simulink model "Discrete_Time_Sim_With_Noise"  (R2024b)
settings: Solver=FixedStepAuto  StartTime=0.0  StopTime=10  FixedStep=0.001  RelTol=1e-3
undefined symbols (not defined in the file or in its folder): DiscIntNeverNeededParam, dspblkCoreblockFVToolHelper, gcbh
libraries: simulink x12, sharedTrackingLibrary x1
(part 1 of 4)
settings Model: Creator=BU  LastModifiedBy=BU

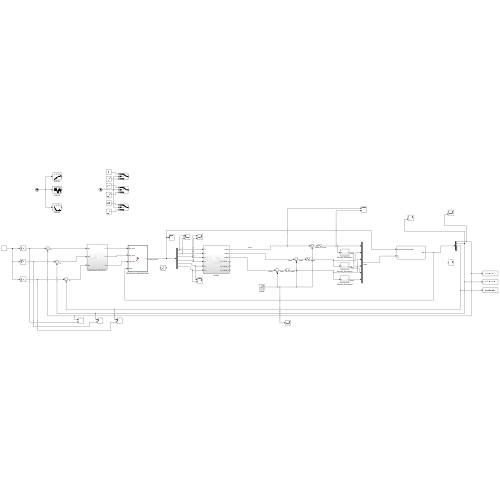
[thumbnail: Simulink's stored preview of the top-level diagram]
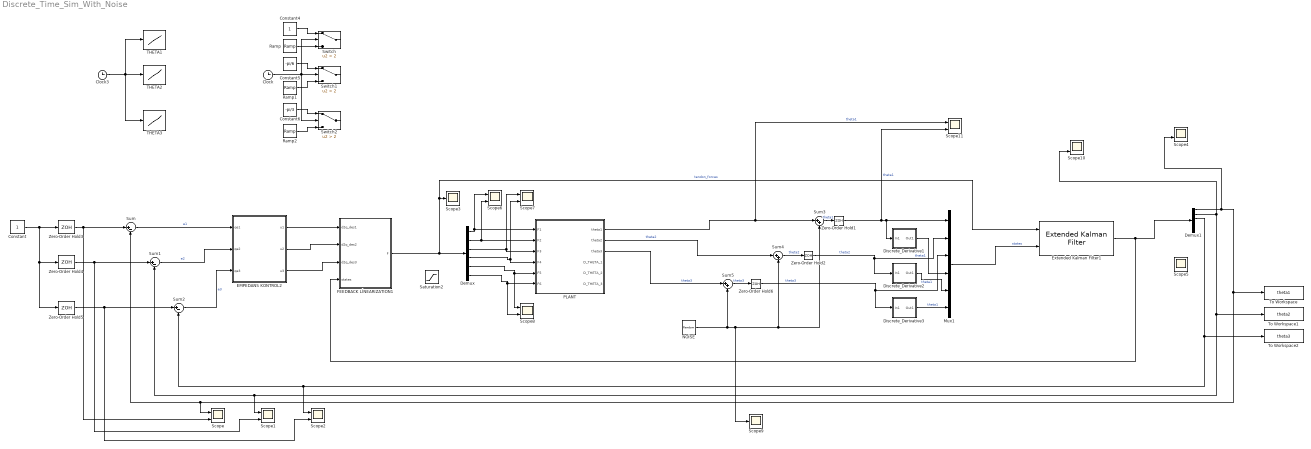
== system Discrete_Time_Sim_With_Noise ==
  Clock : Clock
  Clock3 : Clock
  Constant : Constant
  Constant4 : Constant
  Constant5 : Constant  Value=-pi/6
  Constant6 : Constant  Value=-pi/3
  Demux : Demux  Outputs=6
  Demux1 : Demux  Outputs=6
  Discrete_Derivative1 : Subsystem
  Discrete_Derivative2 : Subsystem
  Discrete_Derivative3 : Subsystem
  EMPEDANS KONTROL2 : Subsystem
  Extended Kalman Filter1 : sharedTrackingLibrary/Extended Kalman Filter  StateTransitionFcn=myStateTransitionFcn  HasStateTransitionJacobianFcn=off  StateTransitionJacobianFcn=0  HasAdditiveProcessNoise=Additive  ProcessNoise=diag([1e-7, 1e-7, 1e-7, 1e-7, 1e-7, 1e-7]);  HasTimeVaryingProcessNoise=off  HasStateTransitionFcnExtraArgument=1  InitialState=[0; 0; 0; 0; 0; 0]  InitialStateCovariance=[1e-6; 1e-6; 1e-6; 1e-6; 1e-6; 1e-6];  MeasurementFcn1=myMeasurementFcn  HasMeasurementJacobianFcn1=off  HasMeasurementEnablePort1=off  HasAdditiveMeasurementNoise1=Additive  MeasurementNoise1=[1e-1; 1e-1; 1e-1; 1e-1; 1e-1; 1e-1];  HasTimeVaryingMeasurementNoise1=off  HasMeasurementFcnExtraArgument1=0  HasMeasurementWrapping1=off  MeasurementFcn2=myMeasurementFcn  HasMeasurementJacobianFcn2=off  HasMeasurementEnablePort2=off  HasAdditiveMeasurementNoise2=Additive  MeasurementNoise2=1  HasTimeVaryingMeasurementNoise2=off  HasMeasurementFcnExtraArgument2=0  HasMeasurementWrapping2=off  MeasurementFcn3=myMeasurementFcn  HasMeasurementJacobianFcn3=off  HasMeasurementEnablePort3=off  HasAdditiveMeasurementNoise3=Additive  MeasurementNoise3=1  HasTimeVaryingMeasurementNoise3=off  HasMeasurementFcnExtraArgument3=0  HasMeasurementWrapping3=off  MeasurementFcn4=myMeasurementFcn  HasMeasurementJacobianFcn4=off  HasMeasurementEnablePort4=off  HasAdditiveMeasurementNoise4=Additive  MeasurementNoise4=1  HasTimeVaryingMeasurementNoise4=off  HasMeasurementFcnExtraArgument4=0  HasMeasurementWrapping4=off  MeasurementFcn5=myMeasurementFcn  HasMeasurementJacobianFcn5=off  HasMeasurementEnablePort5=off  HasAdditiveMeasurementNoise5=Additive  MeasurementNoise5=1  HasTimeVaryingMeasurementNoise5=off  HasMeasurementFcnExtraArgument5=0  HasMeasurementWrapping5=off  EnableMultirate=off  StateTransitionFcnSampleTime=1  MeasurementFcn1SampleTime=1  MeasurementFcn2SampleTime=1  MeasurementFcn3SampleTime=1  MeasurementFcn4SampleTime=1  MeasurementFcn5SampleTime=1  UseCurrentEstimator=on  OutputStateCovariance=off  DataType=double  SampleTime=0.001  NumberOfMeasurements=1
      settings: LibrarySourceBlock=slident/Estimators/Extended Kalman Filter
  FEEDBACK LİNEARIZATION1 : MATLAB Function  TreatAsAtomicUnit=on
  Mux1 : Mux  Inputs=6
  NOİSE : RandomNumber  Variance=6e-6  SampleTime=0.001
  PLANT : Subsystem
  Ramp : simulink/Sources/Ramp  slope=0.5  start=0  InitialOutput=0
  Ramp1 : simulink/Sources/Ramp  slope=-pi/12  start=0  InitialOutput=0
  Ramp2 : simulink/Sources/Ramp  slope=-pi/6  start=0  InitialOutput=0
  Saturation2 : Saturate  UpperLimit=7  LowerLimit=-7
  Scope{,1..2,4,6..8,10..11} (9 alike) : Scope  NumInputPorts=2
  Scope3 : Scope
  Scope5 : Scope
  Scope9 : Scope
  Sum : Sum  Inputs=|+-
  Sum1 : Sum  Inputs=|+-
  Sum2 : Sum  Inputs=|+-
  Sum3 : Sum  Inputs=|++
  Sum4 : Sum  Inputs=|++
  Sum5 : Sum  Inputs=|++
  Switch : Switch  Criteria=u2 > Threshold  Threshold=2  SaturateOnIntegerOverflow=off  InputSameDT=off
  Switch1 : Switch  Criteria=u2 > Threshold  Threshold=2  SaturateOnIntegerOverflow=off  InputSameDT=off
  Switch2 : Switch  Criteria=u2 > Threshold  Threshold=2  SaturateOnIntegerOverflow=off  InputSameDT=off
  THETA1 : Lookup_n-D  NumberOfTableDimensions=1  BreakpointsForDimension1=[0:0.02649:20]  Table="[3.6739403974420595e-17  0.0018373747386941153  0.031104117726482236  0.018742775985835458  0.03582520263747096  0.04592374641467687  0.052359865334245005  0.024058789434421298  0.0371846744639253  0.03766299609142134  0.04053395039223553  0.05419725229851646  0.03858245137367349  0.06940555854089034  0.07349874804657569  0.06036247150750728  0.05603574389361684  0.060203800337469145  0.05742707768917204  0.08742903616174802  0.08902502526928899  0.08910383733839858  0.06737978568977998  0.07977308569010028  0.07440905071740662  0.12217303541401832  0.09094232893350204  0.08904496692572651  0.10747616617119161  0.10938974392795553  0.13962632793396143  0.1083956214534407  0.18488795370701283  0.12080807257958151  0.19198621771937807  0.20053536868258393  0.13958180389913316  0.15159411331235176  0.21221713449958643  0.20813879967607254  0.1559933516267367  0.13924408208160471  0.15768074798413845  0.14168292749125272  0.22330906860945512  0.15983604373103352  0.16455025763473308  0.17031601131911764  0.23328736831901986  0.16908920173142786  0.24223952083150546  0.16676295276355868  0.2460466761118888  0.2427442300425048  0.2486574882599835  0.2524091142547836  0.26497062155526524  0.2686031710582675  0.2501965607304947  0.26676047671265896  0.2643551632848289  0.19274332249535645  0.2738619349890345  0.28220592554301155  0.28811598890932444  0.2734154158379111  0.19658209835701151  0.21602121918276904  0.2672822987058359  0.3286381062553793  0.31016072985042253  0.3333562023023043  0.3206007450683914  0.24027818402917203  0.26820372925417835  0.2671750205501374  0.3316125578789242  0.3426470130069342  0.3512794501726035  0.35378674308527575  0.34906585039886256  0.3602220148407348  0.334007825546644  0.35850389060191834  0.36346154149840965  0.3499372161164522  0.27940999409903805  0.3615110009749353  0.2829285466528819  0.28907124992067035  0.2958562209487426  0.37063784854548126  0.38431676246130947  0.3872502136853321  0.38783712884126237  0.3085945485814749  0.2961223513979233  0.31466855250366454  0.38909946387464134  0.3798718789620668  0.4007313511201461  0.4014257279586968  0.38565996627791466  0.330166531071065  0.33344993261761385  0.3108624823799387  0.3352853086354352  0.40657748147216466  0.34998446799647454  0.3343689689304545  0.4014257279586976  0.4111813198409137  0.3988981447289421  0.4186382947143397  0.40142572795869536  0.41887902047864184  0.4290229802606445  0.41781912282973876  0.41795816369666855  0.43746763932430155  0.41493598188809466  0.43603007682123895  0.41732493944380256  0.34440344919783417  0.42938623750992094  0.45298201367972535  0.4288419913470435  0.3677411229875971  0.43758514195346915  0.3865802197767727  0.3751084506612871  0.44814429494692254  0.3720896409650807  0.4525537516630718  0.45581996404987013  0.46350881524855264  0.3868228290174442  0.46007677244678846  0.47338681502372737  0.4712388980384691  0.4493903916162998  0.4642709337838176  0.4032631026973869  0.4685622431028752  0.3883857325472519  0.46719629998405016  0.4795595869316255  0.41992086739321355  0.3914676248964888  0.40759533432809686  0.48633741377695394  0.503361410251195  0.4837780015498778  0.4884893851013152  0.41753664465676027  0.4085774671942687  0.4315817277722004  0.42719707263790824  0.5026342919632628  0.5125437672769803  0.44002440524952796  0.4333772620748816  0.5105491774179737  0.5281996949991661  0.4886921905584105  0.4282797975188503  0.5173518691902903  0.5238681952025085  0.5278284238409199  0.5288725340894371  0.5416647490392732  0.5149332000522006  0.5502478095136083  0.5462177778009292  0.5402498088439542  0.5286973749476239  0.45219733563073633  0.5333967879492966  0.5410820534657627  0.4704351055583119  0.5421823655200836  0.5559404870228405  0.48551809760352327  0.5480768236319203  0.5574563364291668  0.5719520739146396  0.5718223517553729  0.5747046356092969  0.5591900066960385  0.5579012852080848  0.5530351144405614  0.5664360138663578  0.566709099544408  0.5816224503929176 ...(+11127 chars)];"  InternalRulePriority=Speed  RndMeth=Simplest
  THETA2 : Lookup_n-D  NumberOfTableDimensions=1  BreakpointsForDimension1=[0:0.02649:20]  Table="[0.0  0.03490658503988885  -0.033284041948025575  0.024108973093034097  0.017453292519947913  0.010897133595376871  2.580956827951785e-08  0.05801510497744568  0.04868897935829344  0.05235987755982642  0.060690073963622776  0.03490658503990476  0.06981317007977231  0.024238413989330437  0.014730566219418576  0.05579073535311509  0.06981317007977231  0.06823361310456687  0.08130478950558964  0.028160994381164636  0.03194749988012217  0.034906585039914305  0.08472703296472568  0.07144632904991825  0.08726646259971634  2.580956827951785e-08  0.06981317007977549  0.08192340488382562  0.05235987755983278  0.05540554109194949  2.580956827951785e-08  0.06981317007978505  -0.08840686306026094  0.056301906362856584  -0.08726646259972015  -0.09992958834775573  0.04124423707398681  0.024523948301493594  -0.10278030666584669  -0.08493047048957507  0.0330576678310699  0.07509376311585307  0.044753552033083295  0.08238435334413935  -0.09053757172286077  0.052359877559807325  0.04559052981096805  0.04183361289751157  -0.08806346617828203  0.05457713814060981  -0.10020250825383402  0.06585773908739219  -0.09503207893317432  -0.08382912684246552  -0.0886095062350847  -0.08877482543867116  -0.11289958939038655  -0.11400494326389625  -0.06780086460973182  -0.09787633235095192  -0.08494579017009243  0.07259786120584893  -0.09502044892588707  -0.10858388920763397  -0.11716142564727819  -0.07797060352501026  0.0872664625997125  0.08623656651485352  0.008941650029711387  -0.12003519103250365  -0.07443881028729186  -0.12005690683677152  -0.08711768024630258  0.08609866483557414  0.037707101369440575  0.04564547046169879  -0.08726646259972015  -0.10740555498876758  -0.12175208995592679  -0.12075780610488446  -0.10471975511965279  -0.12431198461645662  -0.06124914974178794  -0.10914281092122118  -0.11751340501827023  -0.08264071659361362  0.06996856329094929  -0.09923579646961392  0.06981317007976753  0.06356008523867811  0.059060910667330074  -0.09563230456995794  -0.120231530929497  -0.1233688014218704  -0.12118747138531023  0.05273873482906122  0.08047001912219476  0.04667516779941028  -0.10697141125366606  -0.08244410112317954  -0.12423265131075169  -0.12217304763960532  -0.0839214967334022  0.03814885382421918  0.034906585039895216  0.08535061346156758  0.039753719555991836  -0.10723463591055922  0.017453292519897023  0.05235987755983278  -0.08726646259972015  -0.10420225604982192  -0.07319022629209936  -0.11164835857706268  -0.06981317007977231  -0.10471975511966554  -0.12268815644386528  -0.09427459346404958  -0.09243646265768085  -0.1304306398657574  -0.07894393826895223  -0.12050390133646655  -0.07656286796138893  0.08061183608047065  -0.08894014674562721  -0.1357335445848138  -0.07816767295833149  0.054119332737865365  -0.08935408926939761  0.02199468753231221  0.05029869437163041  -0.10100975249936778  0.06255747691272129  -0.10489102534646705  -0.10819821457663435  -0.11931485080023811  0.04600742129117378  -0.1061216956455849  -0.1308529653505546  -0.1221730476396035  -0.07202008470981623  -0.099462587755587  0.034906585039895216  -0.10009203093905035  0.07120370686977313  -0.08849603242699301  -0.11159991366826001  0.01842492915558315  0.08166734018060748  0.05474075805682762  -0.10779457600445713  -0.1411952409075954  -0.0946854051550396  -0.10105261328295449  0.052105244970079956  0.0805434765835345  0.039851461664634664  0.05120354563972951  -0.10572128681989593  -0.12333296158987568  0.03422551094635462  0.05191335639712643  -0.10740470199761225  -0.14150127587830474  -0.05235987755982642  0.07865865445022234  -0.090142570581727  -0.10009950108652808  -0.10559245849112399  -0.10486516636439701  -0.12910085175104827  -0.06839935798121312  -0.14041441654823544  -0.12793480610576502  -0.11190815237909614  -0.08442067718491744  0.08121382491144723  -0.08763734115108718  -0.09968809522423466  0.05255504521596442  -0.09395492969943792  -0.12070347296111478  0.0322100128957269  -0.09931879841590988  -0.11511469777161175 ...(+12333 chars)];"  InternalRulePriority=Speed  RndMeth=Simplest
  THETA3 : Lookup_n-D  NumberOfTableDimensions=1  BreakpointsForDimension1=[0:0.02649:20]  Table="[1.4901161157108252e-08  -0.08910383733841787  -0.0327266608183487  -0.12139156541861737  -0.17545154279702416  -0.19644722016959976  -0.19198623130335932  -0.21297358831144533  -0.2429532865017081  -0.2471025063307386  -0.27575694955529145  -0.2636367625378544  -0.282928546652879  -0.29435683650957045  -0.2802155319853704  -0.32559271709994325  -0.3352884242127084  -0.34660356994132824  -0.36562466995402293  -0.3512094795621464  -0.365318620428616  -0.3683565176575177  -0.3964529139337104  -0.4130188025391666  -0.4234749011162723  -0.4014257415426788  -0.4400081793323686  -0.45894769838861765  -0.45654201657006255  -0.47022790411891413  -0.4537856191025084  -0.49236805689220453  -0.41064035600573134  -0.49999589056138904  -0.4363323129985795  -0.4409449844737227  -0.5386185376319574  -0.5426372045326548  -0.4759559707525487  -0.4984541183652786  -0.5730234548965603  -0.6070369268961825  -0.603860027975918  -0.6254930087940876  -0.5254705785853191  -0.6136216492495379  -0.6115665154043974  -0.6223019984352975  -0.5553762763594051  -0.6425453603506759  -0.5521893867963389  -0.6514997123295901  -0.5786202639173261  -0.5865207699386508  -0.5963802950234814  -0.6086932480746661  -0.5971299914234329  -0.608383833312897  -0.6449079478992603  -0.6313963961402045  -0.6506482711532061  -0.7453067279996465  -0.6588070303615892  -0.6535875806338188  -0.6509201075604881  -0.6841370028713132  -0.7725407515151371  -0.8258565612959209  -0.8260026631137608  -0.7496549833411186  -0.7855006339413441  -0.7630780098437462  -0.7919884254602746  -0.8848822095029318  -0.8731428375217765  -0.888779144169965  -0.8203047484373329  -0.8112001111762953  -0.8054860133748054  -0.8177142363984913  -0.8377580409572819  -0.8293219759023509  -0.8748972677429  -0.851499671618741  -0.8480867284181834  -0.8781617377208543  -0.960243795588003  -0.8731404427033367  -0.9636069549306653  -0.9634965733573642  -0.9745090160740592  -0.8945974284335108  -0.8836771159897994  -0.8834732967214486  -0.8862415419139391  -0.9896518141284941  -1.0049109012380764  -0.9983888972810051  -0.9191732295989057  -0.9431996010767902  -0.9222705230472953  -0.9250245035569944  -0.9562369390423859  -1.031540500653129  -1.031581633415354  -1.0594382115993513  -1.0469907902092443  -0.9712946075794223  -1.0481161687941598  -1.067407254768076  -0.9948376736367662  -0.9876574720688799  -1.0151129729746031  -0.9963949906750376  -1.0297442586766548  -1.0122909661567079  -1.0044665246145112  -1.030402876423393  -1.032380048096691  -1.0138953465162475  -1.0515770369368176  -1.0311111688024481  -1.06507371106006  -1.1493269248559512  -1.0647577303419402  -1.0415601086725585  -1.0837126042263305  -1.1636253878230531  -1.0899959847816612  -1.1590664856666466  -1.1758987233904792  -1.0976261208051166  -1.1938653424953358  -1.1068809509341389  -1.1068399740907695  -1.1034121890658484  -1.2007751211861226  -1.1218999476787086  -1.110478720550677  -1.1170107212763702  -1.15404182404396  -1.141479863165707  -1.2235678511347308  -1.1538683755612729  -1.2537142490744457  -1.1815517234744497  -1.170811129180758  -1.2499238987261603  -1.2847130672544596  -1.2826408408222596  -1.1988475862098313  -1.1824709177809345  -1.2181239910921449  -1.2164681665156671  -1.2986732843241466  -1.3181523384751097  -1.309191230394113  -1.316158659234916  -1.2346710461006452  -1.2269688466443822  -1.3207346034131313  -1.3317753056892574  -1.2496291626376115  -1.2331831063381107  -1.2915436464758057  -1.3621497854462936  -1.2911472783457563  -1.2877066738531733  -1.2861739450869882  -1.2879453474622333  -1.276501877025418  -1.3191984680681523  -1.2737713727025661  -1.2822209514323577  -1.2922796362020519  -1.3082146774998995  -1.3973491402793765  -1.3096974265354027  -1.3053319379787212  -1.3956547767714418  -1.3296187080777822  -1.3166282863188619  -1.4078460290163584  -1.338875943733119  -1.3324595571746636  -1.3199035285802887  -1.3240551752124028  -1.323686083948212  -1.3533032032202255  -1.358112045604476 ...(+11743 chars)];"  InternalRulePriority=Speed  RndMeth=Simplest
  To Workspace : ToWorkspace  VariableName=theta1  SaveFormat=Timeseries  SampleTime=-1
  To Workspace1 : ToWorkspace  VariableName=theta2  SaveFormat=Timeseries  SampleTime=-1
  To Workspace2 : ToWorkspace  VariableName=theta3  SaveFormat=Timeseries  SampleTime=-1
  Zero-Order Hold{1..6} (6 alike) : ZeroOrderHold  SampleTime=0.001
  wires:
  Sum/1 -> EMPEDANS KONTROL2/1(qe1)  "e1"
  Sum1/1 -> EMPEDANS KONTROL2/2(qe2)  "e2"
  FEEDBACK LİNEARIZATION1/1(F) -> Extended Kalman Filter1/1, Scope3/1, Demux/1  "tendon_forces"
  Demux/1 -> Scope6/1, PLANT/1(F1)
  Demux/2 -> Scope6/2, PLANT/2(F2)
  Demux/3 -> PLANT/3(F3), Scope7/1
  Demux/4 -> PLANT/4(F4), Scope7/2
  Demux/5 -> Scope8/1, PLANT/5(F5)
  Demux/6 -> Scope8/2, PLANT/6(F6)
  EMPEDANS KONTROL2/3(u3) -> FEEDBACK LİNEARIZATION1/3(d2q_des3)
  EMPEDANS KONTROL2/1(u1) -> FEEDBACK LİNEARIZATION1/1(d2q_des1)
  EMPEDANS KONTROL2/2(u2) -> FEEDBACK LİNEARIZATION1/2(d2q_des2)
  Sum2/1 -> EMPEDANS KONTROL2/3(qe3)  "e3"
  Zero-Order Hold4/1 -> Sum1/1, Scope1/2
  Zero-Order Hold5/1 -> Sum2/1, Scope2/2
  Ramp/1 -> Switch/3
  Constant4/1 -> Switch/1
  Constant5/1 -> Switch1/1
  Ramp1/1 -> Switch1/3
  Constant6/1 -> Switch2/1
  Ramp2/1 -> Switch2/3
  Clock/1 -> Switch2/2, Switch/2, Switch1/2
  Clock3/1 -> THETA3/1, THETA2/1, THETA1/1
  PLANT/3(theta3) -> Sum5/1  "theta3"
  PLANT/2(theta2) -> Sum4/1  "theta2"
  Sum4/1 -> Zero-Order Hold2/1  "theta2"
  Sum3/1 -> Zero-Order Hold1/1  "theta1"
  Zero-Order Hold1/1 -> Scope11/2, Mux1/1, Discrete_Derivative1/1(In1)  "theta1"
  NOİSE/1 -> Scope9/1, Sum3/2, Sum4/2, Sum5/2
  Sum5/1 -> Zero-Order Hold6/1  "theta3"
  PLANT/1(theta1) -> Scope11/1, Sum3/1  "theta1"
  Zero-Order Hold2/1 -> Discrete_Derivative2/1(In1), Mux1/2  "theta2"
  Discrete_Derivative1/1(Out1) -> Mux1/4  "theta1"
  Discrete_Derivative2/1(Out1) -> Mux1/5  "theta1"
  Discrete_Derivative3/1(Out1) -> Mux1/6  "theta1"
  Demux1/3 -> To Workspace2/1, Scope2/1, Sum2/2
  Demux1/1 -> Scope4/2, To Workspace/1, Scope/1, Sum/2
  Demux1/2 -> To Workspace1/1, Scope1/1, Sum1/2, Scope10/2
  Mux1/1 -> Extended Kalman Filter1/2  "states"
  Zero-Order Hold6/1 -> Discrete_Derivative3/1(In1), Mux1/3  "theta3"
  Extended Kalman Filter1/1 -> FEEDBACK LİNEARIZATION1/4(states), Demux1/1
  Zero-Order Hold3/1 -> Sum/1, Scope/2
  Constant/1 -> Zero-Order Hold5/1, Zero-Order Hold4/1, Zero-Order Hold3/1
